simulink model "Ex2_Loadmodelling"  (R2022a)
settings: Solver=ode23tb  StartTime=0.0  StopTime=2  MaxStep=10e-6  RelTol=1e-3  EnableMultiTasking=on
undefined symbols (not defined in the file or in its folder): sigbuilder_block
settings Model: Creator=minothi  LastModifiedBy=thomas
settings SolverCC: AlgebraicLoopSolver=TrustRegion  SolverResetMethod=Robust
settings DataIOCC: LimitDataPoints=on  SaveFormat=Array  SignalLoggingSaveFormat=ModelDataLogs  ReturnWorkspaceOutputs=off
settings OptimizationCC: ExpressionDepthLimit=2147483647  InitFltsAndDblsToZero=on  LifeSpan=inf
settings DebuggingCC: SaveWithParameterizedLinksMsg=none  UnderspecifiedInitializationDetection=Classic  MergeDetectMultiDrivingBlocksExec=none  SignalResolutionControl=TryResolveAllWithWarning  SolverPrmCheckMsg=warning  MultiTaskDSMMsg=warning  MultiTaskCondExecSysMsg=none  FcnCallInpInsideContextMsg=warning  UnconnectedInputMsg=warning  UnconnectedOutputMsg=warning  UnconnectedLineMsg=warning  AllowSymbolicDim=off  StateNameClashWarn=warning  PregeneratedLibrarySubsystemCodeDiagnostic=none  SFUnexpectedBacktrackingDiag=warning  SFNoUnconditionalDefaultTransitionDiag=warning  SFExecutionAtInitializationDiag=none  SFMachineParentedDataDiag=warning  ArithmeticOperatorsInVariantConditions=warning
settings HardwareCC: ProdBitPerPointer=32  ProdBitPerSizeT=32  ProdBitPerPtrDiffT=32  ProdLargestAtomicFloat=None  ProdIntDivRoundTo=Undefined  ProdEndianess=Unspecified  ProdWordSize=32  ProdHWDeviceType=32-bit Generic
settings ModelReferenceCC: PropagateSignalLabelsOutOfModel=off
settings SFSimCC: SimUseLocalCustomCode=off  CustomCodeUndefinedFunction=UseInterfaceOnly  SimTargetLang=C++
settings RTWCC: RTWUseLocalCustomCode=off
settings CodeAppCC: StateflowObjectComments=on
settings GRTTargetCC: TargetFcnLib=ansi_tfl_tmw.mat  TargetLangStandard=C89/C90 (ANSI)  CombineOutputUpdateFcns=off  GRTInterface=on
settings ConfigComp: CovMetricSettings=dw  CovSaveCumulativeToWorkspaceVar=on  CovSaveSingleToWorkspaceVar=on  CovExternalEMLEnable=off
settings SimscapeCC: SimscapeNormalizeSystem=off

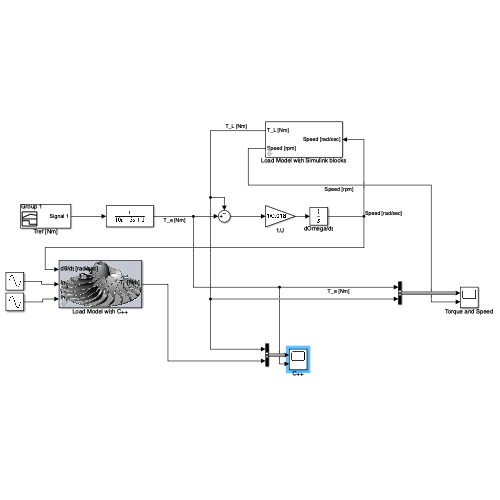
[thumbnail: Simulink's stored preview of the top-level diagram]
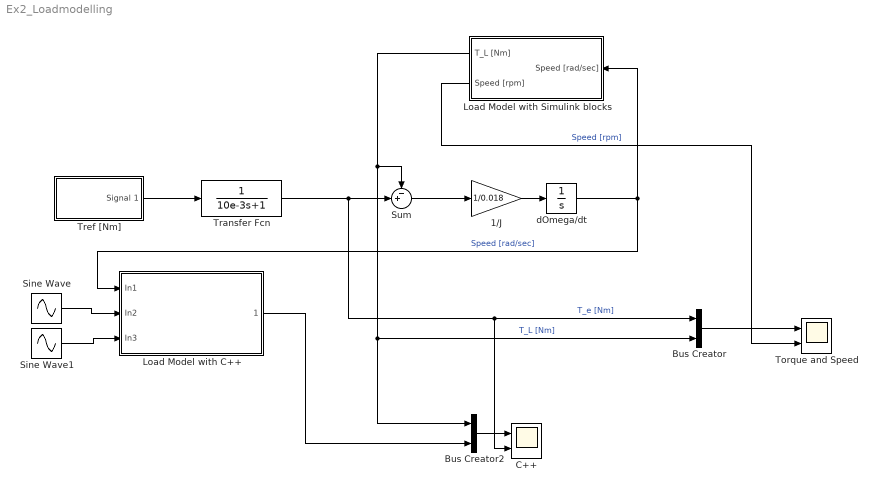
== system Ex2_Loadmodelling ==
  1/J : Gain  Gain=1/0.018
  Bus Creator : BusCreator  Inputs=2
  Bus Creator2 : BusCreator  Inputs=2
  C++ : Scope  NumInputPorts=2
  Load Model with C++ : Subsystem  mask(Model of Mechanical Load){var0=0.1, var1=0.5, var2=0.2, loadSelector=Pump}
      mask prompts: var0 "#0"; var1 "#1"; var2 "#2"; loadSelector "Load Type"
      mask help:
      | This block uses S-Function to implement mechanical load emulator. Input/Output behaviour is described using C/C++ and can be altered by editing the source files "SwLoadEmulator.cpp" and "SwLoadEmulator.hpp".
      |
      | The block has a number of input ports and tunable auxillary mask parameters that you can/need to use when programming certain load characteristics.
      |
      | [Port Name -- C++ name -- data_type -- Description]
      |
      | ----------------- INPUTS -----------------
      | 1)  dTheta / dT -- ActSpeed_rpm -- fp32_t -- Mechanical speed [rpm]
      | 2)  In_0 -- input_sig0 -- fp32_t -- Auxillary signal 0
      | 3)  In_1 -- input_sig1 -- fp32_t -- Auxillary signal 1
      |
      | ----------------- OUTPUTS -----------------
      | 1)  T_L -- m_T_load_Nm -- fp32_t -- Load torque [Nm]
      |
      | ----------------- MASK PARAMETERS -----------------
      | 1)  Auxillary Parameter #0 -- param_var[0] -- fp32_t -- Aux parameter
      | 2)  Auxillary Parameter #1 -- param_var[1] -- fp32_t -- Aux parameter
      | 3)  Auxillary Parameter #2 -- param_var[2] -- fp32_t -- Aux parameter
      mask Help:
      | <h1>TET4120</h1>
      | We can help you! <br> Hello World.
      mask TypeOptions loadSelector: Pump | Electric Vehicle | Ship Propulsion | Wind Power | Hydro Power
      mask DialogControl ParameterGroupVar Prompt: Auxillary Parameters
      mask Display:
      | loadType = get_param(gcb,'loadSelector');
      | switch(loadType)
      |     case 'Pump'
      |         image('graphics/impeller.jpg');
      |     case 'Electric Vehicle'
      |         image('graphics/tesla.jpg')
      |     case 'Ship Propulsion'
      |         image('graphics/marine_vessel.jpg')
      |     case 'Wind Power'
      |         image('graphics/offshore_wind.jpeg')
      |     case 'Hydro Power'
      |         image('graphics/hydro.jpg')
      |     otherwise
      |         % NOP
      | end
      | 
      | port_label('input',1,'d\theta/dt [rad/sec]','texmode','on');
      | port_label('input',2,'In_{0}','texmode','on');
      | port_label('input',3,'In_{1}','texmode','on');
      | port_label('output',1,'T_L [Nm]','texmode','on');
  Load Model with Simulink blocks : Subsystem  mask{k_L=1e-4}
      mask prompts: k_L "kL [Nm/(rad/s)^2]"
      mask DialogControl kL Prompt: Parameters
  Sine Wave : Sin  Amplitude=0.2  Frequency=10  SampleTime=0
  Sine Wave1 : Sin  Amplitude=0.04  Frequency=30  SampleTime=0
  Sum : Sum  Inputs=-+|
  Torque and Speed : Scope  NumInputPorts=2
  Transfer Fcn : TransferFcn  Denominator=[10e-3 1]
  Tref [Nm] : Subsystem  Tag=STV Subsys  LoadFcn=sigbuilder_block('load');  StartFcn=sigbuilder_block('start');  StopFcn=sigbuilder_block('stop');  ClipboardFcn=sigbuilder_block('clipboard');  mask(Sigbuilder block){tuvar=[0:10]}
      mask help: Simulink:masks:SigbuilderBlock_MD
      mask init:
      | if ~strcmp(get_param(bdroot(gcbh),'SimulationStatus'),'stopped') tuvar = sigbuilder_block('maskInit'); end
      settings: CopyFcn=sigbuilder_block('copy');  DeleteFcn=sigbuilder_block('delete');  ModelCloseFcn=sigbuilder_block('modelClose');  PreSaveFcn=sigbuilder_block('preSave');  PauseFcn=sigbuilder_block('pause');  ContinueFcn=sigbuilder_block('continue');  NameChangeFcn=sigbuilder_block('namechange');  OpenFcn=sigbuilder_block('open',[524 331 550.5 400 ]);  CloseFcn=sigbuilder_block('close');
      mask Display: plot(0, 0, 100, 100,[2, 2, 32, 32, 2], [68, 8, 8, 68, 68],[32, 2], [38, 38], [32, 19, 2],[53, 60, 44], [32, 17, 17, 2],[16, 16, 31, 31]);txt = getActiveGroup(gcbh);text(2, 100, txt,'verticalAlignment', 'top');
  dOmega/dt : Integrator
  wires:
  Sum/1 -> 1/J/1
  Transfer Fcn/1 -> C++/2, Bus Creator/1, Sum/2  "T_e [Nm]"
  1/J/1 -> dOmega/dt/1
  Bus Creator/1 -> Torque and Speed/1
  Load Model with Simulink blocks/1(T_L [Nm]) -> Sum/1, Bus Creator2/1, Bus Creator/2  "T_L [Nm]"
  Load Model with Simulink blocks/2(Speed [rpm]) -> Torque and Speed/2  "Speed [rpm]"
  dOmega/dt/1 -> Load Model with C++/1(In1), Load Model with Simulink blocks/1(Speed [rad/sec])  "Speed [rad/sec]"
  Bus Creator2/1 -> C++/1
  Tref [Nm]/1(Signal 1) -> Transfer Fcn/1
  Load Model with C++/1(" ") -> Bus Creator2/2
  Sine Wave/1 -> Load Model with C++/2(In2)
  Sine Wave1/1 -> Load Model with C++/3(In3)

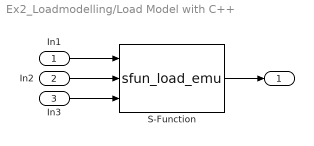
== system Ex2_Loadmodelling/Load Model with C++ ==
  In1 : Inport
  In2 : Inport  Port=2
  In3 : Inport  Port=3
  S-Function : S-Function  FunctionName=sfun_load_emu  Parameters=var0, var1, var2, loadSelector  SFunctionDeploymentMode=off  EnableBusSupport=off
  " " : Outport
  wires:
  In1/1 -> S-Function/1
  In2/1 -> S-Function/2
  S-Function/1 -> " "/1
  In3/1 -> S-Function/3

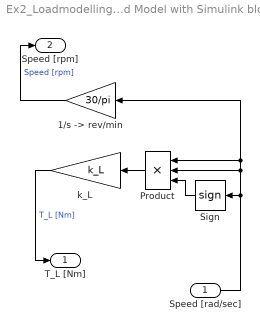
== system Ex2_Loadmodelling/Load Model with Simulink blocks ==
  Speed [rad/sec] : Inport
  "1/s -> rev/min" : Gain  Gain=30/pi
  Product : Product  Inputs=3
  Sign : Signum
  k_L : Gain  Gain=k_L
  T_L [Nm] : Outport
  Speed [rpm] : Outport  Port=2
  wires:
  Product/1 -> k_L/1
  Sign/1 -> Product/3
  k_L/1 -> T_L [Nm]/1  "T_L [Nm]"
  Speed [rad/sec]/1 -> Sign/1, "1/s -> rev/min"/1, Product/1, Product/2
  "1/s -> rev/min"/1 -> Speed [rpm]/1  "Speed [rpm]"

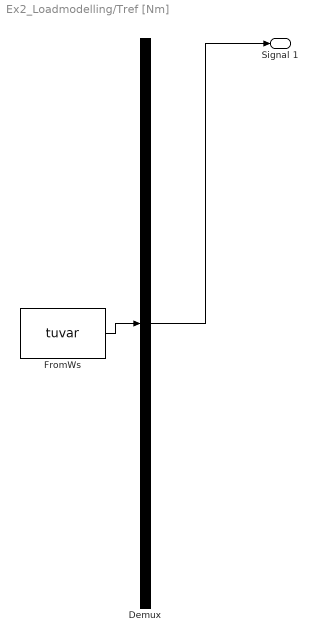
== system Ex2_Loadmodelling/Tref [Nm] ==
  Demux : Demux  Tag=STV Demux  Outputs=1
      settings: DisplayOption=none
  FromWs : FromWorkspace  Tag=STV FromWs  VariableName=tuvar
      SigBuilderData=|
      | common.afterFinalStr = 'Extrapolate'
      | common.sampleTime = 0
      | dataSet.timeRange = [0 2]
      | dataSet.name = 'Group 1'
      | sbobj.Groups.Name = 'Group 1'
      | sbobj.Groups.Signals.Name = 'Signal 1'
      | sbobj.Groups.Signals.XData = [0 0.065 0.065 0.605 0.605 0.805 0.805 1.405 1.405 2]
      | sbobj.Groups.Signals.YData = [0 0 0.595 0.595 0 0 -0.365 -0.365 0 0]
      | sbobj.Groups.TimeRange = [0 2]
  Signal 1 : Outport  Tag=STV Outport
  wires:
  Demux/1 -> Signal 1/1
  FromWs/1 -> Demux/1
